simulink model "forward_converter"  (R2021a)
settings: Solver=VariableStepAuto  StartTime=0.0  StopTime=5  RelTol=1e-3
libraries: spsSeriesRLCBranchLib x4, spsDiodeLib x3, spsVoltageMeasurementLib x2, spsControlledVoltageSourceLib x1, spsIdealSwitchLib x1, spsCurrentMeasurementLib x1, spsLinearTransformerLib x1, spsMosfetLib x1, spsPWMGeneratorDCDCLib x1, msbUtilities x1, spspowerguiLib x1
settings Model: Creator=ACER  LastModifiedBy=ACER

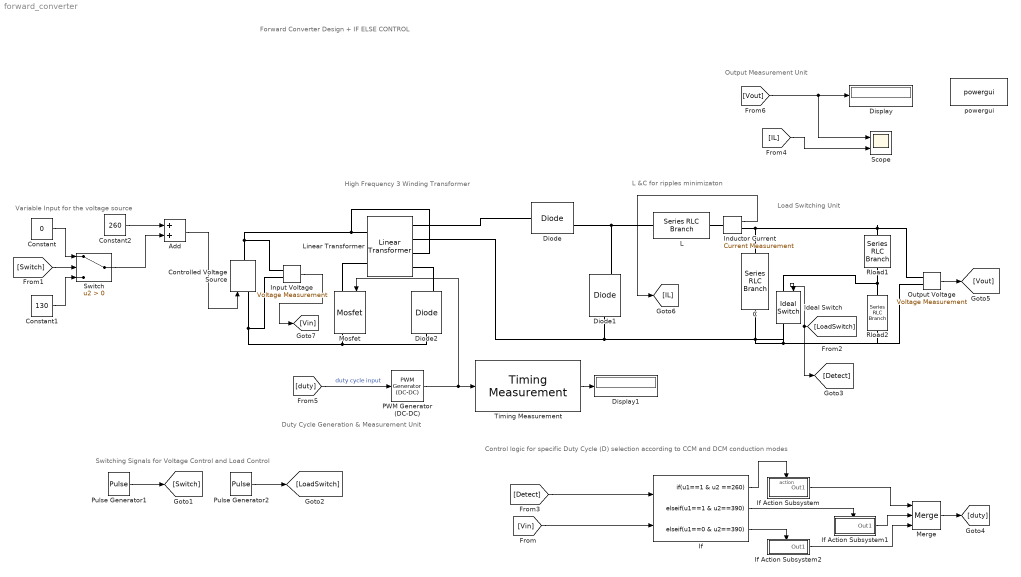
== system forward_converter ==
  note: Forward Converter Design + IF ELSE CONTROL
  note: Output Measurement Unit
  note: Control logic for specific Duty Cycle (D) selection according to CCM and DCM conduction modes
  note: Switching Signals for Voltage Control and Load Control
  note: Load Switching Unit
  note: L &C for ripples minimizaton
  note: High Frequency 3 Winding Transformer
  note: Duty Cycle Generation & Measurement Unit
  note: Variable Input for the voltage source
  Add : Sum
  C : spsSeriesRLCBranchLib/Series RLC Branch  LConnTagsString=__new0  RConnTagsString=__new0  BranchType=C  Resistance=1  Inductance=1e-3  SetiL0=off  InitialCurrent=0  Capacitance=25e-6  Setx0=off  InitialVoltage=0  Measurements=None
  Constant : Constant  Value=0
  Constant1 : Constant  Value=130
  Constant2 : Constant  Value=260
  Controlled Voltage Source : spsControlledVoltageSourceLib/Controlled Voltage Source  Initialize=on  Source_Type=AC  Amplitude=0  Phase=0  Frequency=0  Measurements=None
  Diode : spsDiodeLib/Diode  Ron=0.001  Lon=0  Vf=0.8  IC=0  UseSnubber=0  Rs=500  Cs=250e-9  Measurements=on
  Diode1 : spsDiodeLib/Diode  Ron=0.001  Lon=0  Vf=0.8  IC=0  UseSnubber=0  Rs=500  Cs=250e-9  Measurements=on
  Diode2 : spsDiodeLib/Diode  Ron=0.001  Lon=0  Vf=0.8  IC=0  UseSnubber=0  Rs=500  Cs=250e-9  Measurements=on
  Display : Display
  Display1 : Display
  Ideal Switch : spsIdealSwitchLib/Ideal Switch  Ron=0.001  Lon=0  IC=0  Rs=1e5  Cs=inf  Measurements=on
  If : If  NumInputs=2  IfExpression=u1==1 & u2 ==260  ElseIfExpressions=u1==1 & u2==390, u1==0 & u2==390  ShowElse=off
  If Action Subsystem : Subsystem  TreatAsAtomicUnit=on
  If Action Subsystem1 : Subsystem  TreatAsAtomicUnit=on
  If Action Subsystem2 : Subsystem  TreatAsAtomicUnit=on
  Inductor Current : spsCurrentMeasurementLib/Current Measurement  PhasorSimulation=off  OutputType=Complex  PSBequivalent=0
  Input Voltage : spsVoltageMeasurementLib/Voltage Measurement  PhasorSimulation=off  OutputType=Complex  PSBequivalent=0
  L : spsSeriesRLCBranchLib/Series RLC Branch  LConnTagsString=__new0  RConnTagsString=__new0  BranchType=L  Resistance=1  Inductance=26e-6  SetiL0=off  InitialCurrent=0  Capacitance=1e-6  Setx0=off  InitialVoltage=0  Measurements=None
  Linear Transformer : spsLinearTransformerLib/Linear Transformer  UNITS=pu  NominalPower=[ 100 100e3 ]  winding1="[ 390  0  0]"  winding2="[ 48.75  0  0 ]"  ThreeWindings=on  winding3=[ 390 0 0 ]  RmLm=[ 1.0805e6 2866 ]  Measurements=None  DataType=off
  Merge : Merge  Inputs=3
  Mosfet : spsMosfetLib/Mosfet  Ron=0.1  Lon=0  Rd=0.01  Vfd=0  IC=0  Rs=1e5  Cs=inf  Measurements=on
  Output Voltage : spsVoltageMeasurementLib/Voltage Measurement  PhasorSimulation=off  OutputType=Complex  PSBequivalent=0
  PWM Generator (DC-DC) : spsPWMGeneratorDCDCLib/PWM Generator (DC-DC)  Fsw=100e3  Ts=0
  Pulse Generator1 : DiscretePulseGenerator  PulseType=Time based  Period=4  PulseWidth=25
  Pulse Generator2 : DiscretePulseGenerator  PulseType=Time based  Period=4  PulseWidth=50
  Rload1 : spsSeriesRLCBranchLib/Series RLC Branch  LConnTagsString=__new0  RConnTagsString=__new0  BranchType=R  Resistance=1.125  Inductance=1e-3  SetiL0=off  InitialCurrent=0  Capacitance=1e-6  Setx0=off  InitialVoltage=0  Measurements=None
  Rload2 : spsSeriesRLCBranchLib/Series RLC Branch  LConnTagsString=__new0  RConnTagsString=__new0  BranchType=R  Resistance=10.125  Inductance=1e-3  SetiL0=off  InitialCurrent=0  Capacitance=1e-6  Setx0=off  InitialVoltage=0  Measurements=None
  Scope : Scope  NumInputPorts=2
  Switch : Switch  Criteria=u2 > Threshold
  Timing Measurement : msbUtilities/Timing Measurement  Period=off  Frequency=off  RiseTime=off  FallTime=off  DutyCycle=on  Delay=off  SameRefThreshold=on  GlobalRefThreshold=0  Range=[-1 1]  MeasurementType=80% / 20%  ThresholdMax=0.6  ThresholdMin=-0.6  DcRefThreshold=0  DelayRefThreshold=0  DelayTstThreshold=0
      settings: SourceProductBaseCode=AM
  powergui : spspowerguiLib/powergui  Priority=1  SimulationMode=Continuous  SampleTime=50e-6  frequency=60  Iterations=50  frequencyindice=0  Pbase=100e6  ErrMax=1e-4  UnitsV=kV  UnitsW=MW  buscounter=0  FunctionMessages=off  echomessages=off  EnableUseOfTLC=off  CurrentSourceSwitches=off  DisableSnubberDevices=off  DisableRonSwitches=off  DisableVfSwitches=off  DisplayEquations=off  AutomaticDiscreteSolvers=off  SolverType=Tustin/Backward Euler (TBE)  Interpol=off  ExternalGateDelay=off  methode=off  Ts=100  x0status=blocks  SPID=on  SwTol=0  HookPort=off  NonlinearTolerance=1e-4  nMaxIteration=100  ContinueOnMaxIteration=off  RestoreLinks=warning  ResistiveCurrentMeasurement=off  Frange=[0:2:500]  Ylog=off  Xlog=on  ShowGrid=off  save=off  variable=ZData  structure=0  ZoomFFT=off  StartTime=0.0  cycles=1  DisplayStyle=1  fundamental=60  FreqAxis=off  MaxFrequency=1000  frequencyindicesteady=1  RmsSteady=1  display=off
  wires:
  Pulse Generator1/1 -> [Switch]
  [Switch] -> Switch/2
  Constant/1 -> Switch/1
  Constant1/1 -> Switch/3
  Constant2/1 -> Add/1
  Switch/1 -> Add/2
  Add/1 -> Controlled Voltage Source/1
  Pulse Generator2/1 -> [LoadSwitch]
  [LoadSwitch] -> Ideal Switch/1, [Detect]
  [Detect] -> If/1
  [Vin] -> If/2
  If/1 -> If Action Subsystem/Action
  If/2 -> If Action Subsystem1/Action
  If/3 -> If Action Subsystem2/Action
  If Action Subsystem/1(Out1) -> Merge/1
  If Action Subsystem1/1(Out1) -> Merge/2
  If Action Subsystem2/1(Out1) -> Merge/3
  Merge/1 -> [duty]
  [duty] -> PWM Generator (DC-DC)/1  "duty cycle input"
  Output Voltage/1 -> [Vout]
  [Vout] -> Scope/1, Display/1
  PWM Generator (DC-DC)/1 -> Mosfet/1, Timing Measurement/1
  Timing Measurement/1 -> Display1/1
  Inductor Current/1 -> [IL]
  [IL] -> Scope/2
  Input Voltage/1 -> [Vin]
  connections:
  Controlled Voltage Source/RConn1 -- Input Voltage/LConn1 -- Linear Transformer/RConn3 -- Linear Transformer/LConn1
  Controlled Voltage Source/LConn1 -- Diode2/LConn1 -- Mosfet/RConn1 -- Input Voltage/LConn2
  Diode/LConn1 -- Linear Transformer/RConn1
  L/LConn1 -- Diode1/RConn1 -- Diode/RConn1
  Rload1/LConn1 -- Inductor Current/RConn1 -- C/LConn1 -- Output Voltage/LConn1
  Linear Transformer/RConn2 -- Diode1/LConn1 -- Output Voltage/LConn2 -- Rload2/RConn1 -- Ideal Switch/RConn1 -- C/RConn1
  Mosfet/LConn1 -- Linear Transformer/LConn2
  Diode2/RConn1 -- Linear Transformer/RConn4
  Rload2/LConn1 -- Ideal Switch/LConn1 -- Rload1/RConn1
  Inductor Current/LConn1 -- L/RConn1

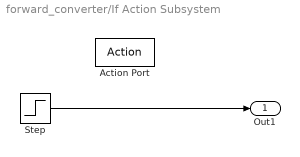
== system forward_converter/If Action Subsystem ==
  Action Port : ActionPort  ActionPortLabel=if(u1==1 & u2 ==260)
  Step : Step  Before=0.4615  After=0.4615  SampleTime=0
  Out1 : Outport
  wires:
  Step/1 -> Out1/1

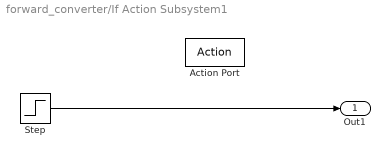
== system forward_converter/If Action Subsystem1 ==
  Action Port : ActionPort  ActionPortLabel=elseif(u1==1 & u2==390)
  Step : Step  Before=0.308  After=0.308  SampleTime=0
  Out1 : Outport
  wires:
  Step/1 -> Out1/1

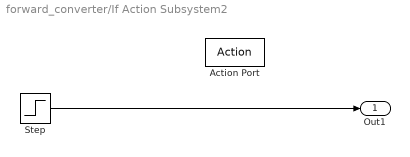
== system forward_converter/If Action Subsystem2 ==
  Action Port : ActionPort  ActionPortLabel=elseif( u1==0 & u2==390)
  Step : Step  Before=0.2512  After=0.2512  SampleTime=0
  Out1 : Outport
  wires:
  Step/1 -> Out1/1
